simulink model "MassaPontoMANSUP_2018b"  (R2024a)
settings: Solver=VariableStepAuto  StartTime=0.0  StopTime=D.Tfim  FixedStep=0.01  MaxStep=0.01  RelTol=1e-3  EnableMultiTasking=on
values from neighbouring files (symbols this model uses):
  C = CondLanc(HORIZONTAL, 15000, 0)    [run_mansup_case.m]
  D = DadosMissil    [run_mansup_case.m]
undefined symbols (not defined in the file or in its folder): m, s
libraries: simulink x12, aerolibatmos2 x3, aerolibasang x2, aerolibconvert x1, aerolibptmass x1, sharedutil x1
settings Model: Creator=Administrador  LastModifiedBy=mathe
settings SolverCC: AlgebraicLoopSolver=TrustRegion
settings DataIOCC: LimitDataPoints=on  SaveFormat=Array  SignalLoggingSaveFormat=ModelDataLogs  ReturnWorkspaceOutputs=off
settings OptimizationCC: ExpressionDepthLimit=2147483647  LifeSpan=inf
settings DebuggingCC: UnderspecifiedInitializationDetection=Classic  MergeDetectMultiDrivingBlocksExec=none  SolverPrmCheckMsg=warning  FcnCallInpInsideContextMsg=warning  UnconnectedInputMsg=warning  UnconnectedOutputMsg=warning  UnconnectedLineMsg=warning  StateNameClashWarn=warning  SFUnexpectedBacktrackingDiag=warning  SFNoUnconditionalDefaultTransitionDiag=warning  SFExecutionAtInitializationDiag=none  ArithmeticOperatorsInVariantConditions=warning
settings HardwareCC: ProdBitPerPointer=32  ProdBitPerSizeT=32  ProdBitPerPtrDiffT=32  ProdLargestAtomicFloat=None  ProdIntDivRoundTo=Undefined  ProdEndianess=Unspecified  ProdWordSize=32  ProdHWDeviceType=32-bit Generic
settings ModelReferenceCC: EnableRefExpFcnMdlSchedulingChecks=on  PropagateSignalLabelsOutOfModel=off
settings SFSimCC: SimUseLocalCustomCode=off  CustomCodeUndefinedFunction=UseInterfaceOnly
settings RTWCC: RTWUseLocalCustomCode=off  GPUComputeCapability=3.5
settings CodeAppCC: StateflowObjectComments=on
settings GRTTargetCC: TargetLangStandard=C89/C90 (ANSI)  CombineOutputUpdateFcns=off  GRTInterface=on
settings ConfigComp: CovMetricSettings=dw  CovSaveCumulativeToWorkspaceVar=on  CovSaveSingleToWorkspaceVar=on  CovExternalEMLEnable=off  CovSFcnEnable=off

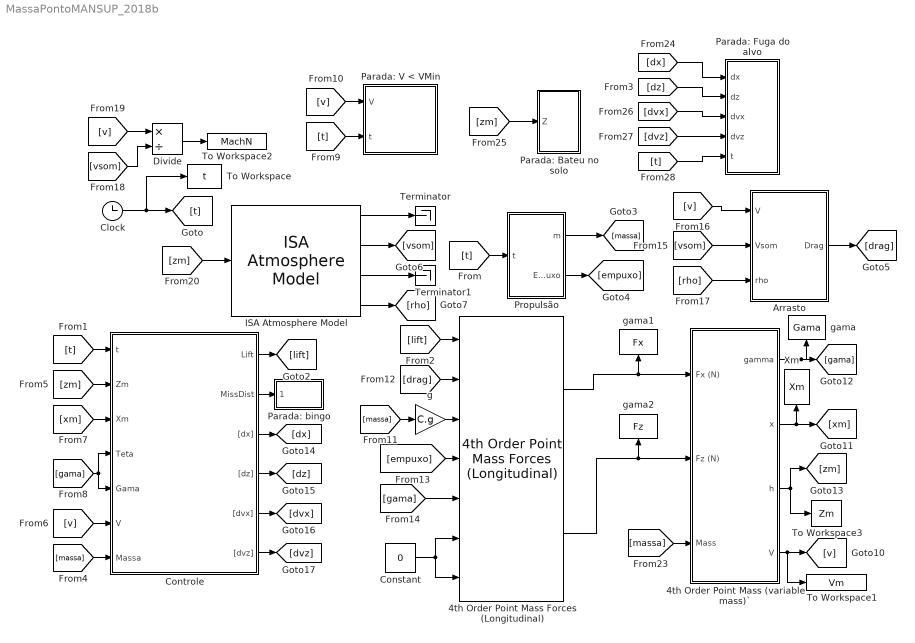
== system MassaPontoMANSUP_2018b ==
  4th Order Point Mass (variable mass)` : Subsystem
  4th Order Point Mass Forces (Longitudinal) : aerolibptmass/4th Order Point Mass Forces (Longitudinal)
  Arrasto : Subsystem
  Clock : Clock
  Constant : Constant  Value=0
  Controle : Subsystem
  Divide : Product  Inputs=*/
  ISA Atmosphere Model : aerolibatmos2/ISA Atmosphere Model  useExtended=off  action=Warning  custom=off  viscosityOut=off  g=9.80665  gamma=1.4  R=287.0531  L=0.0065  h_trop=11000  h_strat=20000  rho0=1.225  P0=101325  T0=288.15  h0=0  S=110.4  Tref=273.15  muref=1.716e-5
  Parada: Bateu no solo : Subsystem
  Parada: Fuga do alvo : Subsystem
  Parada: V < VMin : Subsystem
  Parada: bingo : Subsystem
  "Propulsão " : Subsystem
  Terminator : Terminator
  Terminator1 : Terminator
  To Workspace : ToWorkspace  VariableName=t  SampleTime=-1
  To Workspace1 : ToWorkspace  VariableName=Vm  SaveFormat=Timeseries  SampleTime=-1
  To Workspace2 : ToWorkspace  VariableName=MachN  SaveFormat=Timeseries  SampleTime=-1
  To Workspace3 : ToWorkspace  VariableName=Zm  SaveFormat=Timeseries  SampleTime=-1
  Xm : ToWorkspace  VariableName=Xm  SaveFormat=Timeseries  SampleTime=-1
  g : Gain  Gain=C.g
  gama : ToWorkspace  VariableName=Gama  SaveFormat=Timeseries  SampleTime=-1
  gama1 : ToWorkspace  VariableName=Fx  SaveFormat=Timeseries  SampleTime=-1
  gama2 : ToWorkspace  VariableName=Fz  SaveFormat=Timeseries  SampleTime=-1
  wires:
  Clock/1 -> To Workspace/1, [t]
  Constant/1 -> 4th Order Point Mass Forces (Longitudinal)/7, 4th Order Point Mass Forces (Longitudinal)/6
  4th Order Point Mass (variable mass)`/1(gamma) -> [gama], gama/1
  4th Order Point Mass (variable mass)`/2(x) -> [xm], Xm/1
  4th Order Point Mass (variable mass)`/3(h) -> To Workspace3/1, [zm]
  ISA Atmosphere Model/3 -> Terminator1/1
  4th Order Point Mass (variable mass)`/4(V) -> [v], To Workspace1/1
  Controle/2(MissDist) -> Parada: bingo/1(MissDist)
  [t] -> "Propulsão "/1(t)
  [t] -> Controle/1(t)
  Controle/1(Lift) -> [lift]
  [lift] -> 4th Order Point Mass Forces (Longitudinal)/1
  [dz] -> Parada: Fuga do alvo/2(dz)
  [massa] -> Controle/7(Massa)
  [zm] -> Controle/2(Zm)
  [v] -> Controle/6(V)
  [xm] -> Controle/3(Xm)
  [gama] -> Controle/4(Teta), Controle/5(Gama)
  [t] -> Parada: V < VMin/2(t)
  [v] -> Parada: V < VMin/1(V)
  "Propulsão "/1(m) -> [massa]
  "Propulsão "/2(Empuxo) -> [empuxo]
  [massa] -> g/1
  [drag] -> 4th Order Point Mass Forces (Longitudinal)/2
  [empuxo] -> 4th Order Point Mass Forces (Longitudinal)/4
  [gama] -> 4th Order Point Mass Forces (Longitudinal)/5
  Arrasto/1(Drag) -> [drag]
  [vsom] -> Arrasto/2(Vsom)
  [v] -> Arrasto/1(V)
  [rho] -> Arrasto/3(rho)
  Divide/1 -> To Workspace2/1
  [v] -> Divide/1
  [vsom] -> Divide/2
  ISA Atmosphere Model/2 -> [vsom]
  ISA Atmosphere Model/4 -> [rho]
  ISA Atmosphere Model/1 -> Terminator/1
  [zm] -> ISA Atmosphere Model/1
  4th Order Point Mass Forces (Longitudinal)/1 -> gama1/1, 4th Order Point Mass (variable mass)`/1(Fx (N))
  4th Order Point Mass Forces (Longitudinal)/2 -> gama2/1, 4th Order Point Mass (variable mass)`/2(Fz (N))
  [massa] -> 4th Order Point Mass (variable mass)`/3(Mass)
  [dx] -> Parada: Fuga do alvo/1(dx)
  [zm] -> Parada: Bateu no solo/1(Z)
  g/1 -> 4th Order Point Mass Forces (Longitudinal)/3
  [dvx] -> Parada: Fuga do alvo/3(dvx)
  [dvz] -> Parada: Fuga do alvo/4(dvz)
  [t] -> Parada: Fuga do alvo/5(t)
  Controle/6("[dvz]") -> [dvz]
  Controle/5("[dvx]") -> [dvx]
  Controle/4("[dz]") -> [dz]
  Controle/3("[dx]") -> [dx]

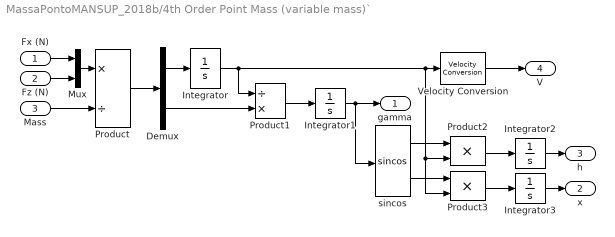
== system MassaPontoMANSUP_2018b/4th Order Point Mass (variable mass)` ==
  Fx (N) : Inport
  Fz (N) : Inport  Port=2
  Mass : Inport  Port=3
  Demux : Demux  Outputs=2
  Integrator : Integrator  InitialCondition=C.V0
  Integrator1 : Integrator  InitialCondition=C.Gama0
  Integrator2 : Integrator  InitialCondition=C.Z0m
  Integrator3 : Integrator  InitialCondition=C.X0m
  Mux : Mux  Inputs=2
  Product : Product  Inputs=*/  SaturateOnIntegerOverflow=on  OutDataTypeStr=Inherit: Same as first input
  Product1 : Product  Inputs=/*  SaturateOnIntegerOverflow=on  OutDataTypeStr=Inherit: Same as first input
  Product2 : Product  SaturateOnIntegerOverflow=on  OutDataTypeStr=Inherit: Same as first input
  Product3 : Product  SaturateOnIntegerOverflow=on  OutDataTypeStr=Inherit: Same as first input
  Velocity Conversion : aerolibconvert/Velocity Conversion  IU=m/s  OU=m/s
  sincos : Trigonometry  Operator=sincos
  gamma : Outport  VectorParamsAs1DForOutWhenUnconnected=off
  x : Outport  Port=2  VectorParamsAs1DForOutWhenUnconnected=off
  h : Outport  Port=3  VectorParamsAs1DForOutWhenUnconnected=off
  V : Outport  Port=4  VectorParamsAs1DForOutWhenUnconnected=off
  wires:
  Product3/1 -> Integrator3/1
  Integrator3/1 -> x/1
  Integrator2/1 -> h/1
  Integrator1/1 -> gamma/1, sincos/1
  Product2/1 -> Integrator2/1
  sincos/2 -> Product3/1
  sincos/1 -> Product2/1
  Product1/1 -> Integrator1/1
  Demux/1 -> Integrator/1
  Mux/1 -> Product/1
  Fz (N)/1 -> Mux/2
  Fx (N)/1 -> Mux/1
  Product/1 -> Demux/1
  Integrator/1 -> Product1/1, Product3/2, Product2/2, Velocity Conversion/1
  Velocity Conversion/1 -> V/1
  Mass/1 -> Product/2
  Demux/2 -> Product1/2

== system MassaPontoMANSUP_2018b/Arrasto ==
  V : Inport
  Vsom : Inport  Port=2
  rho : Inport  Port=3
  Arrasto1 : Product  Inputs=*****
  CD : Lookup_n-D  NumberOfTableDimensions=1  BreakpointsForDimension1=D.Cd(:,1)  Table=D.Cd(:,2)  ExtrapMethod=Clip  RndMeth=Simplest
  Product1 : Product  Inputs=*/  RndMeth=Zero
  To Workspace5 : ToWorkspace  VariableName=FDrag  SaveFormat=Timeseries  SampleTime=-1
  q : Constant  Value=0.5*D.SRef
  Drag : Outport  VectorParamsAs1DForOutWhenUnconnected=off
  wires:
  Vsom/1 -> Product1/2
  q/1 -> Arrasto1/4
  Arrasto1/1 -> To Workspace5/1, Drag/1
  rho/1 -> Arrasto1/5
  V/1 -> Arrasto1/3, Arrasto1/2, Product1/1
  Product1/1 -> CD/1
  CD/1 -> Arrasto1/1

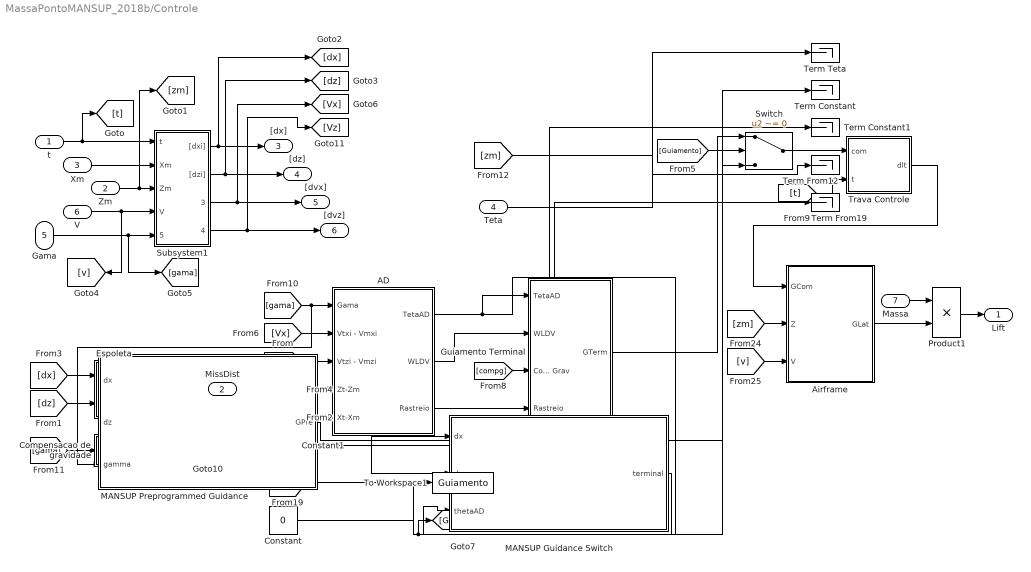
== system MassaPontoMANSUP_2018b/Controle ==
  t : Inport
  Zm : Inport  Port=2
  Xm : Inport  Port=3
  Teta : Inport  Port=4
  Gama : Inport  Port=5
  V : Inport  Port=6
  Massa : Inport  Port=7
  AD : Subsystem
  Airframe : Subsystem
  Compensacao de gravidade : Subsystem
  Constant : Constant  Value=0
  Constant1 : Constant
  Espoleta : Subsystem
  Guiamento Terminal : Subsystem
  MANSUP Guidance Switch : Subsystem
  MANSUP Preprogrammed Guidance : Subsystem
  Product1 : Product  Inputs=**  RndMeth=Zero
  Subsystem1 : Subsystem
  Switch : Switch  Criteria=u2 ~= 0  ZeroCross=off  SaturateOnIntegerOverflow=off  InputSameDT=off
  Term Constant : Terminator
  Term Constant1 : Terminator
  Term From12 : Terminator
  Term From19 : Terminator
  Term Teta : Terminator
  To Workspace1 : ToWorkspace  VariableName=Guiamento  SaveFormat=Timeseries  SampleTime=-1
  Trava Controle : Subsystem
  Lift : Outport  VectorParamsAs1DForOutWhenUnconnected=off
  MissDist : Outport  Port=2  VectorParamsAs1DForOutWhenUnconnected=off
  "[dx]" : Outport  Port=3  VectorParamsAs1DForOutWhenUnconnected=off
  "[dz]" : Outport  Port=4  VectorParamsAs1DForOutWhenUnconnected=off
  "[dvx]" : Outport  Port=5  VectorParamsAs1DForOutWhenUnconnected=off
  "[dvz]" : Outport  Port=6  VectorParamsAs1DForOutWhenUnconnected=off
  wires:
  Espoleta/1(MissDist) -> MissDist/1
  [dx] -> Espoleta/1(delta X)
  Zm/1 -> [zm], Subsystem1/3(Zm)
  [dz] -> Espoleta/2(delta Z)
  V/1 -> Subsystem1/4(V), [v]
  [gama] -> AD/1(Gama), MANSUP Preprogrammed Guidance/3(gamma)
  Gama/1 -> [gama], Subsystem1/5("gama ")
  [gama] -> Compensacao de gravidade/1(gama)
  Compensacao de gravidade/1(Out1) -> [compg]
  AD/1(TetaAD) -> Guiamento Terminal/1(TetaAD), MANSUP Guidance Switch/3(thetaAD)
  AD/2(WLDV) -> Guiamento Terminal/2(WLDV)
  Guiamento Terminal/1(GTerm) -> Switch/1
  t/1 -> [t], Subsystem1/1(t)
  Xm/1 -> Subsystem1/2(Xm)
  Subsystem1/1("[dxi]") -> "[dx]"/1, [dx]
  Subsystem1/2("[dzi]") -> [dz], "[dz]"/1
  [dx] -> AD/5(Xt-Xm), MANSUP Guidance Switch/1(dx), MANSUP Preprogrammed Guidance/1(dx)
  [dz] -> AD/4(Zt-Zm), MANSUP Guidance Switch/2(dz), MANSUP Preprogrammed Guidance/2(dz)
  Subsystem1/4("[dvzi]") -> "[dvz]"/1, [Vz]
  [Vx] -> AD/2(Vtxi - Vmxi)
  [Vz] -> AD/3(Vtzi - Vmzi)
  Subsystem1/3("[dvxi]") -> "[dvx]"/1, [Vx]
  [Guiamento] -> Switch/2
  Massa/1 -> Product1/1
  Airframe/1(GLat) -> Product1/2
  [v] -> Airframe/3(V)
  [zm] -> Airframe/2(Z)
  AD/3(Rastreio) -> Guiamento Terminal/4(Rastreio)
  [compg] -> Guiamento Terminal/3(Comp Grav)
  Switch/1 -> Trava Controle/1(com)
  Trava Controle/1(dlt) -> Airframe/1(GCom)
  Product1/1 -> Lift/1
  [t] -> Trava Controle/2(t)
  MANSUP Preprogrammed Guidance/1(GPre) -> Switch/3
  MANSUP Guidance Switch/1(terminal) -> [Guiamento], To Workspace1/1
  Teta/1 -> Term Teta/1
  Constant/1 -> Term Constant/1
  Constant1/1 -> Term Constant1/1
  [zm] -> Term From12/1
  [t] -> Term From19/1

== system MassaPontoMANSUP_2018b/Parada: Bateu no solo ==
  Z : Inport
  Compare To Zero : simulink/Logic and Bit Operations/Compare To Zero  relop=<=  OutDataTypeStr=boolean  ZeroCross=off
  Compare To Zero1 : simulink/Logic and Bit Operations/Compare To Zero  relop=<=  OutDataTypeStr=boolean  ZeroCross=off
  Constant : Constant  Value=C.Plano
  Logical Operator : Logic  AllPortsSameDT=off  OutDataTypeStr=boolean
  Stop Simulation : Stop
  To Workspace10 : ToWorkspace  VariableName=Stop_Queda  SampleTime=-1
  wires:
  Z/1 -> Compare To Zero/1
  Compare To Zero/1 -> Logical Operator/1
  Logical Operator/1 -> To Workspace10/1, Stop Simulation/1
  Constant/1 -> Compare To Zero1/1
  Compare To Zero1/1 -> Logical Operator/2

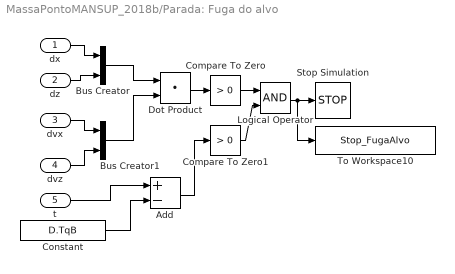
== system MassaPontoMANSUP_2018b/Parada: Fuga do alvo ==
  dx : Inport
  dz : Inport  Port=2
  dvx : Inport  Port=3
  dvz : Inport  Port=4
  t : Inport  Port=5
  Add : Sum  Inputs=+-
  Bus Creator : BusCreator  Inputs=2
  Bus Creator1 : BusCreator  Inputs=2
  Compare To Zero : simulink/Logic and Bit Operations/Compare To Zero  relop=>  OutDataTypeStr=boolean  ZeroCross=off
  Compare To Zero1 : simulink/Logic and Bit Operations/Compare To Zero  relop=>  OutDataTypeStr=boolean  ZeroCross=off
  Constant : Constant  Value=D.TqB
  Dot Product : DotProduct  OutDataTypeStr=Inherit: Inherit via internal rule
  Logical Operator : Logic  AllPortsSameDT=off  OutDataTypeStr=boolean
  Stop Simulation : Stop
  To Workspace10 : ToWorkspace  VariableName=Stop_FugaAlvo  SampleTime=-1
  wires:
  dx/1 -> Bus Creator/1
  dz/1 -> Bus Creator/2
  dvx/1 -> Bus Creator1/1
  dvz/1 -> Bus Creator1/2
  Bus Creator/1 -> Dot Product/1
  Bus Creator1/1 -> Dot Product/2
  Dot Product/1 -> Compare To Zero/1
  Compare To Zero/1 -> Logical Operator/1
  Logical Operator/1 -> To Workspace10/1, Stop Simulation/1
  t/1 -> Add/1
  Add/1 -> Compare To Zero1/1
  Compare To Zero1/1 -> Logical Operator/2
  Constant/1 -> Add/2

== system MassaPontoMANSUP_2018b/Parada: V < VMin ==
  V : Inport
  t : Inport  Port=2
  Compare To Constant : simulink/Logic and Bit Operations/Compare To Constant  relop=<=  const=D.VMin  OutDataTypeStr=boolean
  Compare To Constant1 : simulink/Logic and Bit Operations/Compare To Constant  relop=>=  const=D.TqB  OutDataTypeStr=boolean
  Logical Operator1 : Logic  AllPortsSameDT=off  OutDataTypeStr=boolean
  Stop Simulation2 : Stop
  To Workspace9 : ToWorkspace  VariableName=Stop_VMin  SampleTime=-1
  wires:
  t/1 -> Compare To Constant1/1
  V/1 -> Compare To Constant/1
  Compare To Constant1/1 -> Logical Operator1/2
  Compare To Constant/1 -> Logical Operator1/1
  Logical Operator1/1 -> To Workspace9/1, Stop Simulation2/1

== system MassaPontoMANSUP_2018b/Parada: bingo ==
  MissDist : Inport
  Compare To Constant : simulink/Logic and Bit Operations/Compare To Constant  relop=<=  const=D.REspoleta  OutDataTypeStr=boolean  ZeroCross=off
      link override Constant: Value=D.REspoleta
  Stop Simulation1 : Stop
  To Workspace8 : ToWorkspace  VariableName=Bingo  SampleTime=-1
  wires:
  MissDist/1 -> Compare To Constant/1
  Compare To Constant/1 -> Stop Simulation1/1, To Workspace8/1

== system MassaPontoMANSUP_2018b/Propulsão  ==
  t : Inport
  Empuxo x t : Lookup_n-D  NumberOfTableDimensions=1  BreakpointsForDimension1=D.VProp(:,1)  Table=D.VProp(:,2)  ExtrapMethod=Clip  UseLastTableValue=on  RndMeth=Simplest
  Massa final : Constant  Value=D.Mf
  Sum : Sum  Inputs=|++
  To Workspace6 : ToWorkspace  VariableName=Thrust  SaveFormat=Timeseries  SampleTime=-1
  To Workspace7 : ToWorkspace  VariableName=Massa  SaveFormat=Timeseries  SampleTime=-1
  mprop x t : Lookup_n-D  NumberOfTableDimensions=1  BreakpointsForDimension1=D.VProp(:,1)  Table=D.VProp(:,3)  ExtrapMethod=Clip  UseLastTableValue=on  RndMeth=Simplest
  m : Outport  VectorParamsAs1DForOutWhenUnconnected=off
  Empuxo : Outport  Port=2  VectorParamsAs1DForOutWhenUnconnected=off
  wires:
  Massa final/1 -> Sum/2
  Empuxo x t/1 -> Empuxo/1, To Workspace6/1
  mprop x t/1 -> Sum/1
  t/1 -> Empuxo x t/1, mprop x t/1
  Sum/1 -> m/1, To Workspace7/1

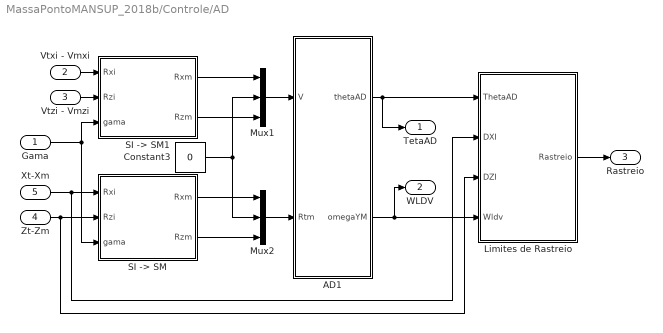
== system MassaPontoMANSUP_2018b/Controle/AD ==
  Gama : Inport
  Vtxi - Vmxi : Inport  Port=2
  Vtzi - Vmzi : Inport  Port=3
  Zt-Zm : Inport  Port=4
  Xt-Xm : Inport  Port=5
  AD1 : Subsystem
  Constant3 : Constant  Value=0
  "Limites de Rastreio " : Subsystem
  Mux1 : Mux  Inputs=3
  Mux2 : Mux  Inputs=3
  "SI -> SM" : Subsystem
  "SI -> SM1" : Subsystem
  TetaAD : Outport  VectorParamsAs1DForOutWhenUnconnected=off
  WLDV : Outport  Port=2  VectorParamsAs1DForOutWhenUnconnected=off
  Rastreio : Outport  Port=3  VectorParamsAs1DForOutWhenUnconnected=off
  wires:
  Zt-Zm/1 -> "Limites de Rastreio "/3(DZI), "SI -> SM"/2(Rzi)
  Gama/1 -> "SI -> SM"/3(gama), "SI -> SM1"/3(gama)
  "SI -> SM"/1(Rxm) -> Mux2/1
  "SI -> SM"/2(Rzm) -> Mux2/3
  Mux2/1 -> AD1/2(Rtm)
  Mux1/1 -> AD1/1(V)
  Vtxi - Vmxi/1 -> "SI -> SM1"/1("Rxi ")
  Vtzi - Vmzi/1 -> "SI -> SM1"/2(Rzi)
  "SI -> SM1"/1(Rxm) -> Mux1/1
  "SI -> SM1"/2(Rzm) -> Mux1/3
  Constant3/1 -> Mux2/2, Mux1/2
  Xt-Xm/1 -> "Limites de Rastreio "/2(DXI), "SI -> SM"/1("Rxi ")
  AD1/1(thetaAD) -> "Limites de Rastreio "/1(ThetaAD), TetaAD/1
  AD1/2(omegaYM) -> "Limites de Rastreio "/4(Wldv), WLDV/1
  "Limites de Rastreio "/1(Rastreio) -> Rastreio/1

== system MassaPontoMANSUP_2018b/Controle/Airframe ==
  GCom : Inport
  Z : Inport  Port=2
  V : Inport  Port=3
  Airframe : TransferFcn  Numerator=[D.wn^2]  Denominator=[1 2*D.qsi*D.wn D.wn^2]
  Limite de Manobra : Subsystem
  To Workspace4 : ToWorkspace  VariableName=GLat  SaveFormat=Timeseries  SampleTime=-1
  gcmd : ToWorkspace  VariableName=GCom  SaveFormat=Timeseries  SampleTime=-1
  GLat : Outport  VectorParamsAs1DForOutWhenUnconnected=off
  wires:
  Airframe/1 -> Limite de Manobra/3(g com)
  GCom/1 -> Airframe/1, gcmd/1
  Limite de Manobra/1(g limitado) -> To Workspace4/1, GLat/1
  V/1 -> Limite de Manobra/2(V)
  Z/1 -> Limite de Manobra/1(Z)

== system MassaPontoMANSUP_2018b/Controle/Compensacao de gravidade ==
  gama : Inport
  Constant : Constant  Value=C.Plano
  Constant1 : Constant  Value=0
  Product : Product  RndMeth=Zero
  Switch : Switch  Criteria=u2 > Threshold  ZeroCross=off  SaturateOnIntegerOverflow=off  InputSameDT=off
  To Workspace4 : ToWorkspace  VariableName=GComp  SaveFormat=Timeseries  SampleTime=-1
  Trigonometric Function1 : Trigonometry  Operator=cos
  g : Constant  Value=C.g
  Out1 : Outport  VectorParamsAs1DForOutWhenUnconnected=off
  wires:
  gama/1 -> Trigonometric Function1/1
  g/1 -> Product/2
  Trigonometric Function1/1 -> Product/1
  Product/1 -> Switch/3
  Constant/1 -> Switch/2
  Constant1/1 -> Switch/1
  Switch/1 -> To Workspace4/1, Out1/1

== system MassaPontoMANSUP_2018b/Controle/Espoleta ==
  delta X : Inport
  delta Z : Inport  Port=2
  Math Function : Math  Operator=square  SignedPower=on
  Math Function1 : Math  Operator=square  SignedPower=on
  Sqrt : Sqrt
  Sum3 : Sum
  To Workspace3 : ToWorkspace  VariableName=MissDist  SaveFormat=Timeseries  SampleTime=-1
  MissDist : Outport  VectorParamsAs1DForOutWhenUnconnected=off
  wires:
  delta Z/1 -> Math Function1/1
  Sqrt/1 -> MissDist/1, To Workspace3/1
  delta X/1 -> Math Function/1
  Sum3/1 -> Sqrt/1
  Math Function1/1 -> Sum3/2
  Math Function/1 -> Sum3/1

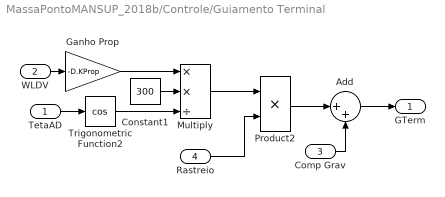
== system MassaPontoMANSUP_2018b/Controle/Guiamento Terminal ==
  TetaAD : Inport
  WLDV : Inport  Port=2
  Comp Grav : Inport  Port=3
  Rastreio : Inport  Port=4
  Add : Sum  Inputs=|++
  Constant1 : Constant  Value=300
  Ganho Prop : Gain  Gain=-D.KProp
  Multiply : Product  Inputs=**/
  Product2 : Product  Inputs=**  RndMeth=Zero
  Trigonometric Function2 : Trigonometry  Operator=cos
  GTerm : Outport  VectorParamsAs1DForOutWhenUnconnected=off
  wires:
  TetaAD/1 -> Trigonometric Function2/1
  WLDV/1 -> Ganho Prop/1
  Ganho Prop/1 -> Multiply/1
  Trigonometric Function2/1 -> Multiply/3
  Constant1/1 -> Multiply/2
  Rastreio/1 -> Product2/2
  Comp Grav/1 -> Add/2
  Multiply/1 -> Product2/1
  Add/1 -> GTerm/1
  Product2/1 -> Add/1

== system MassaPontoMANSUP_2018b/Controle/MANSUP Guidance Switch ==
  dx : Inport
  dz : Inport  Port=2
  thetaAD : Inport  Port=3
  Mux : Mux  Inputs=3
  Terminal logic : Fcn  Expr=(sqrt(u(1)^2+u(2)^2)<=C.TerminalRange)*(abs(u(3))<=D.ThetaADmax)
  terminal : Outport
  wires:
  dx/1 -> Mux/1
  dz/1 -> Mux/2
  thetaAD/1 -> Mux/3
  Mux/1 -> Terminal logic/1
  Terminal logic/1 -> terminal/1

== system MassaPontoMANSUP_2018b/Controle/MANSUP Preprogrammed Guidance ==
  dx : Inport
  dz : Inport  Port=2
  gamma : Inport  Port=3
  Limit : Saturate  UpperLimit=D.AcelLatMax  LowerLimit=-D.AcelLatMax
  Mux : Mux  Inputs=3
  Turn command : Fcn  Expr=D.KPreTurn*(atan2(u(2),u(1))-u(3))
  GPre : Outport
  wires:
  dx/1 -> Mux/1
  dz/1 -> Mux/2
  gamma/1 -> Mux/3
  Mux/1 -> Turn command/1
  Turn command/1 -> Limit/1
  Limit/1 -> GPre/1

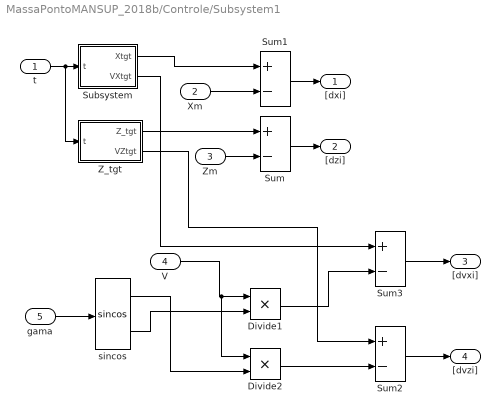
== system MassaPontoMANSUP_2018b/Controle/Subsystem1 ==
  t : Inport
  Xm : Inport  Port=2
  Zm : Inport  Port=3
  V : Inport  Port=4
  "gama " : Inport  Port=5
  Divide1 : Product  Inputs=**
  Divide2 : Product  Inputs=**
  Subsystem : Subsystem
  Sum{,1..3} (4 alike) : Sum  Inputs=+-
  Z_tgt : Subsystem
  sincos : Trigonometry  Operator=sincos
  "[dxi]" : Outport  VectorParamsAs1DForOutWhenUnconnected=off
  "[dzi]" : Outport  Port=2  VectorParamsAs1DForOutWhenUnconnected=off
  "[dvxi]" : Outport  Port=3  VectorParamsAs1DForOutWhenUnconnected=off
  "[dvzi]" : Outport  Port=4  VectorParamsAs1DForOutWhenUnconnected=off
  wires:
  Sum/1 -> "[dzi]"/1
  Zm/1 -> Sum/2
  Sum1/1 -> "[dxi]"/1
  t/1 -> Z_tgt/1(t), Subsystem/1(t)
  Xm/1 -> Sum1/2
  Subsystem/1(Xtgt) -> Sum1/1
  Z_tgt/1(Z_tgt) -> Sum/1
  V/1 -> Divide2/1, Divide1/1
  sincos/2 -> Divide1/2
  "gama "/1 -> sincos/1
  sincos/1 -> Divide2/2
  Divide1/1 -> Sum3/2
  Subsystem/2(VXtgt) -> Sum3/1
  Z_tgt/2(VZtgt) -> Sum2/1
  Divide2/1 -> Sum2/2
  Sum3/1 -> "[dvxi]"/1
  Sum2/1 -> "[dvzi]"/1

== system MassaPontoMANSUP_2018b/Controle/Trava Controle ==
  com : Inport
  t : Inport  Port=2
  Switch1 : Switch  Criteria=u2 > Threshold  Threshold=D.TTrav  ZeroCross=off  SaturateOnIntegerOverflow=off  InputSameDT=off
  c : Constant  Value=0
  dlt : Outport  VectorParamsAs1DForOutWhenUnconnected=off
  wires:
  com/1 -> Switch1/1
  Switch1/1 -> dlt/1
  t/1 -> Switch1/2
  c/1 -> Switch1/3

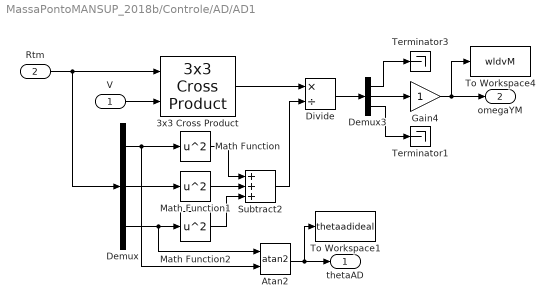
== system MassaPontoMANSUP_2018b/Controle/AD/AD1 ==
  V : Inport
  Rtm : Inport  Port=2
  3x3 Cross Product : sharedutil/3x3 Cross Product  aMode=aMode
  Atan2 : Trigonometry  Operator=atan2
  Demux : Demux  Outputs=3
  Demux3 : Demux  Outputs=3
  Divide : Product  Inputs=*/
  Gain4 : Gain
  Math Function : Math  Operator=square  SignedPower=on
  Math Function1 : Math  Operator=square  SignedPower=on
  Math Function2 : Math  Operator=square  SignedPower=on
  Subtract2 : Sum  Inputs=+++
  Terminator1 : Terminator
  Terminator3 : Terminator
  To Workspace1 : ToWorkspace  VariableName=thetaadideal  SaveFormat=Timeseries  SampleTime=-1
  To Workspace4 : ToWorkspace  VariableName=wldvM  SaveFormat=Timeseries  SampleTime=-1
  thetaAD : Outport  VectorParamsAs1DForOutWhenUnconnected=off
  omegaYM : Outport  Port=2  VectorParamsAs1DForOutWhenUnconnected=off
  wires:
  3x3 Cross Product/1 -> Divide/1
  Demux/2 -> Math Function1/1
  Rtm/1 -> 3x3 Cross Product/1, Demux/1
  Math Function1/1 -> Subtract2/2
  Math Function/1 -> Subtract2/1
  Math Function2/1 -> Subtract2/3
  Subtract2/1 -> Divide/2
  Divide/1 -> Demux3/1
  Demux/1 -> Atan2/2, Math Function/1
  Demux3/1 -> Terminator3/1
  Demux3/3 -> Terminator1/1
  V/1 -> 3x3 Cross Product/2
  Demux3/2 -> Gain4/1
  Gain4/1 -> omegaYM/1, To Workspace4/1
  Demux/3 -> Math Function2/1, Atan2/1
  Atan2/1 -> thetaAD/1, To Workspace1/1

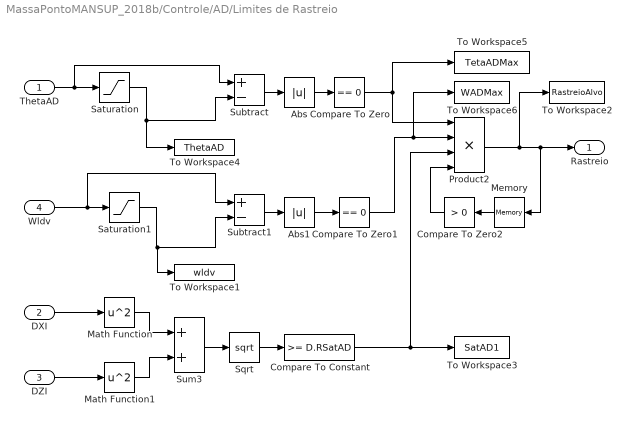
== system MassaPontoMANSUP_2018b/Controle/AD/Limites de Rastreio  ==
  ThetaAD : Inport
  DXI : Inport  Port=2
  DZI : Inport  Port=3
  Wldv : Inport  Port=4
  Abs : Abs  SaturateOnIntegerOverflow=off
  Abs1 : Abs  SaturateOnIntegerOverflow=off
  Compare To Constant : simulink/Logic and Bit Operations/Compare To Constant  relop=>=  const=D.RSatAD  OutDataTypeStr=boolean
  Compare To Zero : simulink/Logic and Bit Operations/Compare To Zero  relop===  OutDataTypeStr=boolean
  Compare To Zero1 : simulink/Logic and Bit Operations/Compare To Zero  relop===  OutDataTypeStr=boolean
  Compare To Zero2 : simulink/Logic and Bit Operations/Compare To Zero  relop=>  OutDataTypeStr=boolean
  Math Function : Math  Operator=square  SignedPower=on
  Math Function1 : Math  Operator=square  SignedPower=on
  Memory : Memory  InitialCondition=1
  Product2 : Product  Inputs=****  RndMeth=Zero
  Saturation : Saturate  UpperLimit=D.ThetaADmax  LowerLimit=-D.ThetaADmax
  Saturation1 : Saturate  UpperLimit=D.OmegaADmax  LowerLimit=-D.OmegaADmax
  Sqrt : Sqrt
  Subtract : Sum  Inputs=+-
  Subtract1 : Sum  Inputs=+-
  Sum3 : Sum
  To Workspace1 : ToWorkspace  VariableName=wldv  SaveFormat=Timeseries  SampleTime=-1
  To Workspace2 : ToWorkspace  VariableName=RastreioAlvo  SaveFormat=Timeseries  SampleTime=-1
  To Workspace3 : ToWorkspace  VariableName=SatAD1  SaveFormat=Timeseries  SampleTime=-1
  To Workspace4 : ToWorkspace  VariableName=ThetaAD  SaveFormat=Timeseries  SampleTime=-1
  To Workspace5 : ToWorkspace  VariableName=TetaADMax  SaveFormat=Timeseries  SampleTime=-1
  To Workspace6 : ToWorkspace  VariableName=WADMax  SaveFormat=Timeseries  SampleTime=-1
  Rastreio : Outport  VectorParamsAs1DForOutWhenUnconnected=off
  wires:
  ThetaAD/1 -> Saturation/1, Subtract/1
  Abs/1 -> Compare To Zero/1
  Abs1/1 -> Compare To Zero1/1
  DXI/1 -> Math Function/1
  Product2/1 -> To Workspace2/1, Rastreio/1, Memory/1
  Saturation/1 -> To Workspace4/1, Subtract/2
  Wldv/1 -> Subtract1/1, Saturation1/1
  Compare To Zero1/1 -> To Workspace6/1, Product2/2
  Compare To Zero/1 -> To Workspace5/1, Product2/1
  DZI/1 -> Math Function1/1
  Subtract/1 -> Abs/1
  Compare To Zero2/1 -> Product2/4
  Memory/1 -> Compare To Zero2/1
  Subtract1/1 -> Abs1/1
  Saturation1/1 -> To Workspace1/1, Subtract1/2
  Sum3/1 -> Sqrt/1
  Math Function/1 -> Sum3/1
  Math Function1/1 -> Sum3/2
  Sqrt/1 -> Compare To Constant/1
  Compare To Constant/1 -> Product2/3, To Workspace3/1

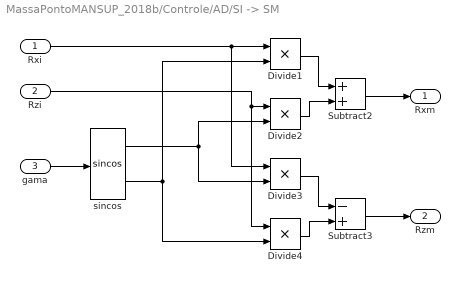
== system MassaPontoMANSUP_2018b/Controle/AD/SI -> SM ==
  "Rxi " : Inport
  Rzi : Inport  Port=2
  gama : Inport  Port=3
  Divide{1..4} (4 alike) : Product  Inputs=**
  Subtract2 : Sum
  Subtract3 : Sum  Inputs=-+
  sincos : Trigonometry  Operator=sincos
  Rxm : Outport  VectorParamsAs1DForOutWhenUnconnected=off
  Rzm : Outport  Port=2  VectorParamsAs1DForOutWhenUnconnected=off
  wires:
  Divide2/1 -> Subtract2/2
  Divide1/1 -> Subtract2/1
  Rzi/1 -> Divide4/1, Divide2/1
  "Rxi "/1 -> Divide3/1, Divide1/1
  sincos/1 -> Divide2/2, Divide3/2
  Divide4/1 -> Subtract3/2
  sincos/2 -> Divide1/2, Divide4/2
  Divide3/1 -> Subtract3/1
  gama/1 -> sincos/1
  Subtract2/1 -> Rxm/1
  Subtract3/1 -> Rzm/1

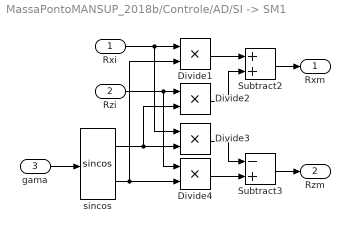
== system MassaPontoMANSUP_2018b/Controle/AD/SI -> SM1 ==
  "Rxi " : Inport
  Rzi : Inport  Port=2
  gama : Inport  Port=3
  Divide{1..4} (4 alike) : Product  Inputs=**
  Subtract2 : Sum
  Subtract3 : Sum  Inputs=-+
  sincos : Trigonometry  Operator=sincos
  Rxm : Outport  VectorParamsAs1DForOutWhenUnconnected=off
  Rzm : Outport  Port=2  VectorParamsAs1DForOutWhenUnconnected=off
  wires:
  Divide2/1 -> Subtract2/2
  Divide1/1 -> Subtract2/1
  Rzi/1 -> Divide4/1, Divide2/1
  "Rxi "/1 -> Divide3/1, Divide1/1
  sincos/1 -> Divide3/2, Divide2/2
  Divide4/1 -> Subtract3/2
  sincos/2 -> Divide4/2, Divide1/2
  Divide3/1 -> Subtract3/1
  gama/1 -> sincos/1
  Subtract2/1 -> Rxm/1
  Subtract3/1 -> Rzm/1

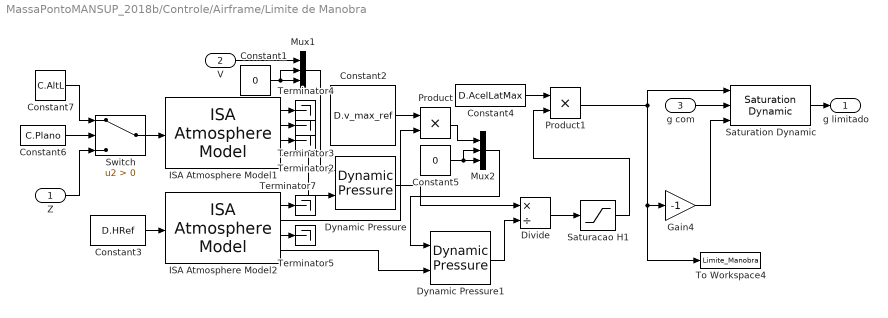
== system MassaPontoMANSUP_2018b/Controle/Airframe/Limite de Manobra ==
  Z : Inport
  V : Inport  Port=2
  g com : Inport  Port=3
  Constant1 : Constant  Value=0
  Constant2 : Constant  Value=D.v_max_ref
  Constant3 : Constant  Value=D.HRef
  Constant4 : Constant  Value=D.AcelLatMax
  Constant5 : Constant  Value=0
  Constant6 : Constant  Value=C.Plano
  Constant7 : Constant  Value=C.AltL
  Divide : Product  Inputs=*/
  Dynamic Pressure : aerolibasang/Dynamic Pressure
  Dynamic Pressure1 : aerolibasang/Dynamic Pressure
  Gain4 : Gain  Gain=-1
  ISA Atmosphere Model1 : aerolibatmos2/ISA Atmosphere Model  useExtended=off  action=Warning  custom=off  viscosityOut=off  g=9.80665  gamma=1.4  R=287.0531  L=0.0065  h_trop=11000  h_strat=20000  rho0=1.225  P0=101325  T0=288.15  h0=0  S=110.4  Tref=273.15  muref=1.716e-5
  ISA Atmosphere Model2 : aerolibatmos2/ISA Atmosphere Model  useExtended=off  action=Warning  custom=off  viscosityOut=off  g=9.80665  gamma=1.4  R=287.0531  L=0.0065  h_trop=11000  h_strat=20000  rho0=1.225  P0=101325  T0=288.15  h0=0  S=110.4  Tref=273.15  muref=1.716e-5
  Mux1 : Mux  Inputs=3
  Mux2 : Mux  Inputs=3
  Product : Product
  Product1 : Product
  Saturacao H1 : Saturate  UpperLimit=1  LowerLimit=0
  Saturation Dynamic : simulink/Discontinuities/Saturation Dynamic  OutMin=[]  OutMax=[]  OutDataTypeStr=Inherit: Same as second input  OutDataType=fixdt(1, 16)  OutScaling=2^-10  DoSatur=off
  Switch : Switch  Criteria=u2 > Threshold  SaturateOnIntegerOverflow=off  InputSameDT=off
  Terminator{2..5,7} (5 alike) : Terminator
  To Workspace4 : ToWorkspace  VariableName=Limite_Manobra  SaveFormat=Timeseries  SampleTime=-1
  g limitado : Outport  VectorParamsAs1DForOutWhenUnconnected=off
  wires:
  Z/1 -> Switch/3
  Saturacao H1/1 -> Product1/2
  ISA Atmosphere Model1/2 -> Terminator3/1
  g com/1 -> Saturation Dynamic/2
  Dynamic Pressure/1 -> Divide/1
  Dynamic Pressure1/1 -> Divide/2
  Switch/1 -> ISA Atmosphere Model1/1
  ISA Atmosphere Model2/4 -> Dynamic Pressure1/2
  Constant4/1 -> Product1/1
  ISA Atmosphere Model1/1 -> Terminator4/1
  ISA Atmosphere Model1/3 -> Terminator2/1
  Constant7/1 -> Switch/1
  Mux1/1 -> Dynamic Pressure/1
  Constant6/1 -> Switch/2
  Mux2/1 -> Dynamic Pressure1/1
  Gain4/1 -> Saturation Dynamic/3
  Product/1 -> Mux2/1
  Divide/1 -> Saturacao H1/1
  Saturation Dynamic/1 -> g limitado/1
  V/1 -> Mux1/1
  ISA Atmosphere Model2/1 -> Terminator7/1
  Constant5/1 -> Mux2/2, Mux2/3
  Constant2/1 -> Product/1
  ISA Atmosphere Model2/2 -> Product/2
  ISA Atmosphere Model2/3 -> Terminator5/1
  Product1/1 -> Gain4/1, To Workspace4/1, Saturation Dynamic/1
  ISA Atmosphere Model1/4 -> Dynamic Pressure/2
  Constant1/1 -> Mux1/3, Mux1/2
  Constant3/1 -> ISA Atmosphere Model2/1

== system MassaPontoMANSUP_2018b/Controle/Subsystem1/Subsystem ==
  t : Inport
  Product3 : Product  Inputs=**  RndMeth=Zero
  Sum : Sum  Inputs=|++
  To Workspace2 : ToWorkspace  VariableName=XTgt  SaveFormat=Timeseries  SampleTime=-1
  VxTgt : Constant  Value=C.VxTgt
  X alvo : Constant  Value=C.X0Tgt
  Xtgt : Outport  VectorParamsAs1DForOutWhenUnconnected=off
  VXtgt : Outport  Port=2  VectorParamsAs1DForOutWhenUnconnected=off
  wires:
  t/1 -> Product3/1
  VxTgt/1 -> VXtgt/1, Product3/2
  X alvo/1 -> Sum/2
  Product3/1 -> Sum/1
  Sum/1 -> To Workspace2/1, Xtgt/1

== system MassaPontoMANSUP_2018b/Controle/Subsystem1/Z_tgt ==
  t : Inport
  " " : Sum  Inputs=+|+
  4 : ToWorkspace  VariableName=ZTgt  SaveFormat=Timeseries  SampleTime=-1
  Product2 : Product  Inputs=**  RndMeth=Zero
  VzTgt : Constant  Value=C.VzTgt
  Z inicial alvo : Constant  Value=C.Z0Tgt
  Z_tgt : Outport  VectorParamsAs1DForOutWhenUnconnected=off
  VZtgt : Outport  Port=2  VectorParamsAs1DForOutWhenUnconnected=off
  wires:
  t/1 -> Product2/2
  " "/1 -> Z_tgt/1, 4/1
  VzTgt/1 -> VZtgt/1, Product2/1
  Product2/1 -> " "/2
  Z inicial alvo/1 -> " "/1
